simulink model "mp62s"  (R2021a)
settings: Solver=VariableStepAuto  StartTime=0.0  StopTime=10.0  MaxStep=1e-3  RelTol=1e-4
values from neighbouring files (symbols this model uses):
  A = [0 1; -k/mass-(4*C_magnetic*Ib^2)/(mass*gap^3) -c/mass]    [ex4.m]    (also in mp62.m = [-2 -3;-1 -4]; od.m = [0 1; -k/m-(4*C_magnetic*Ib^2)/(m*gap^3) -c/m])
  B = [0;(4*C_magnetic*Ib)/(mass*gap^2)]    [ex4.m]    (also in mp62.m = [0 1]'; od.m = [0;(4*C_magnetic*Ib)/(m*gap^2)])
  C = 0.0157    [ex2_1.m]    (also in ex3.m = 3.73e-06; ex4.m = [1 0]; mp62.m = [1 0]; od.m = [1 0;0 0])
  Cf = eye(2)    [mp62.m]
  L = acker(A',C',P)'    [mp62.m]
  X0 = [1;-2]    [mp62.m]
  X0hat = [0;0]    [mp62.m]
settings Model: Creator=dell  LastModifiedBy=dell

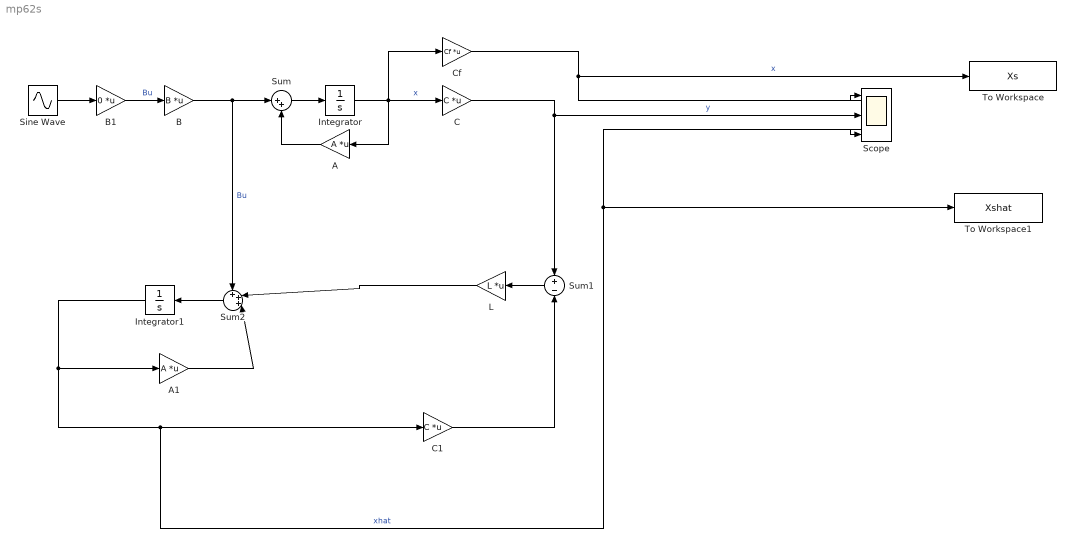
== system mp62s ==
  A : Gain  Gain=A  Multiplication=Matrix(K*u) (u vector)
  A1 : Gain  Gain=A  Multiplication=Matrix(K*u) (u vector)
  B : Gain  Gain=B  Multiplication=Matrix(K*u) (u vector)
  B1 : Gain  Gain=0  Multiplication=Matrix(K*u) (u vector)
  C : Gain  Gain=C  Multiplication=Matrix(K*u) (u vector)
  C1 : Gain  Gain=C  Multiplication=Matrix(K*u) (u vector)
  Cf : Gain  Gain=Cf  Multiplication=Matrix(K*u) (u vector)
  Integrator : Integrator  InitialCondition=X0
  Integrator1 : Integrator  InitialCondition=X0hat
  L : Gain  Gain=L  Multiplication=Matrix(K*u) (u vector)
  Scope : Scope  NumInputPorts=3
  Sine Wave : Sin  Amplitude=10  Frequency=20  SampleTime=0
  Sum : Sum  Inputs=|++
  Sum1 : Sum  Inputs=+|-
  Sum2 : Sum  Inputs=+++|
  To Workspace : ToWorkspace  VariableName=Xs  SaveFormat=Structure With Time  SampleTime=-1
  To Workspace1 : ToWorkspace  VariableName=Xshat  SaveFormat=Structure With Time  SampleTime=-1
  wires:
  Sum/1 -> Integrator/1
  Integrator/1 -> Cf/1, C/1, A/1  "x"
  A/1 -> Sum/2
  B/1 -> Sum2/1, Sum/1  "Bu"
  Sine Wave/1 -> B1/1
  Cf/1 -> To Workspace/1, Scope/1  "x"
  C/1 -> Sum1/1, Scope/2  "y"
  C1/1 -> Sum1/2
  Sum1/1 -> L/1
  L/1 -> Sum2/2
  Integrator1/1 -> Scope/3, To Workspace1/1, C1/1, A1/1  "xhat"
  A1/1 -> Sum2/3
  Sum2/1 -> Integrator1/1
  B1/1 -> B/1  "Bu"
